simulink model "mracsim"  (R2022a)
settings: Solver=VariableStepAuto  StartTime=0.0  StopTime=100  RelTol=1e-3
undefined symbols (not defined in the file): A, Am, B, Bm, Cm, Dm, Gr, Gx, kr, kx
settings Model: Creator=Joseph  LastModifiedBy=Joseph

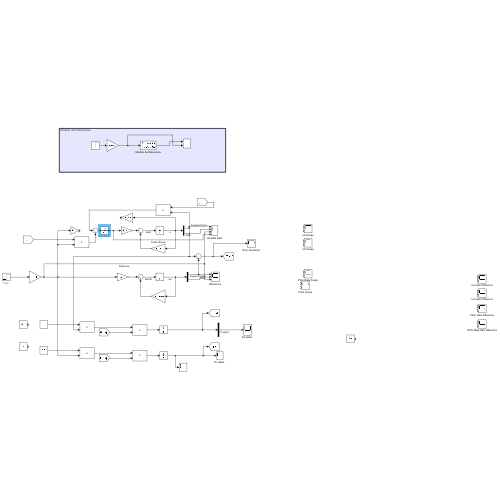
[thumbnail: Simulink's stored preview of the top-level diagram]
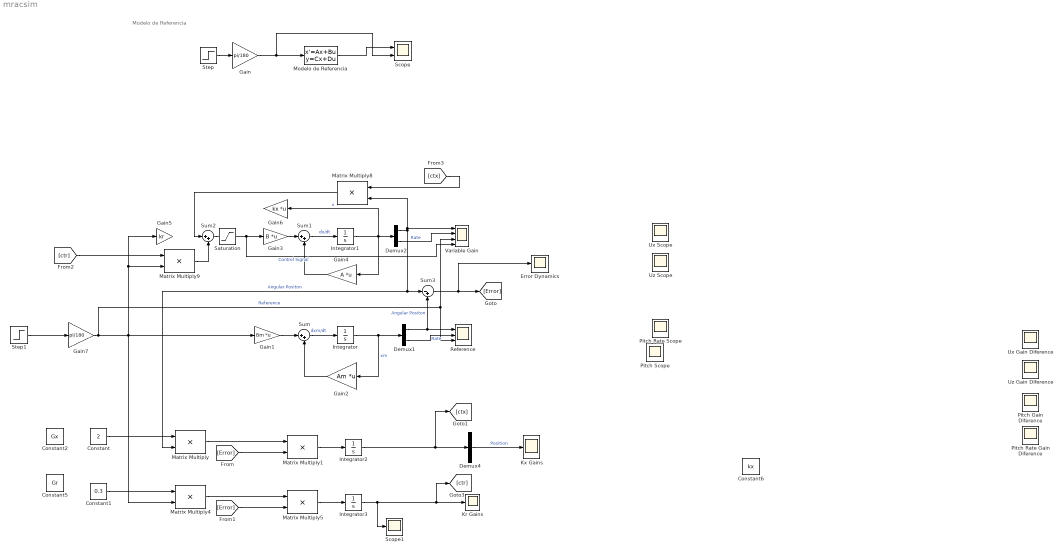
== system mracsim ==
  note: Modelo de Referencia
  Constant : Constant  Value=2
  Constant1 : Constant  Value=0.3
  Constant2 : Constant  Value=Gx
  Constant5 : Constant  Value=Gr
  Constant6 : Constant  Value=kx
  Demux1 : Demux  Outputs=2
  Demux2 : Demux  Outputs=2
  Demux4 : Demux  Outputs=1
  Error Dynamics : Scope
  Gain : Gain  Gain=pi/180
  Gain1 : Gain  Gain=Bm  Multiplication=Matrix(K*u)
  Gain2 : Gain  Gain=Am  Multiplication=Matrix(K*u) (u vector)
  Gain3 : Gain  Gain=B  Multiplication=Matrix(K*u)
  Gain4 : Gain  Gain=A  Multiplication=Matrix(K*u) (u vector)
  Gain5 : Gain  Gain=kr
  Gain6 : Gain  Gain=kx  Multiplication=Matrix(K*u) (u vector)
  Gain7 : Gain  Gain=pi/180
  Integrator{,1..3} (4 alike) : Integrator  ZeroCross=off
  "Kr Gains " : Scope
  "Kx Gains " : Scope
  Matrix Multiply{,1,4..5,8..9} (6 alike) : Product
  Modelo de Referencia : StateSpace  A=Am  B=Bm  C=Cm  D=Dm  InitialCondition=0
  Pitch Gain Diference : Scope  NumInputPorts=2
  Pitch Rate Gain Diference : Scope  NumInputPorts=2
  Pitch Rate Scope : Scope  NumInputPorts=2
  Pitch Scope : Scope  NumInputPorts=2
  Reference : Scope  NumInputPorts=3
  Saturation : Saturate  UpperLimit=9  LowerLimit=0  ZeroCross=off
  Scope : Scope  NumInputPorts=2
  Scope1 : Scope
  Step : Step  Time=0  After=60  SampleTime=0  ZeroCross=off
  Step1 : Step  Time=0  After=60  SampleTime=0  ZeroCross=off
  Sum : Sum  Inputs=|++
  Sum1 : Sum  Inputs=|++
  Sum2 : Sum  Inputs=|++
  Sum3 : Sum  Inputs=|-+
  Ux Gain Diference : Scope  NumInputPorts=2
  Ux Scope : Scope  NumInputPorts=2
  Uz Gain Diference : Scope  NumInputPorts=2
  Uz Scope : Scope  NumInputPorts=2
  Variable Gain : Scope  NumInputPorts=4
  wires:
  Step/1 -> Gain/1
  Gain/1 -> Scope/2, Modelo de Referencia/1
  Modelo de Referencia/1 -> Scope/1
  [ctr] -> Matrix Multiply9/1
  Integrator/1 -> Demux1/1, Gain2/1  "xm"
  [ctx] -> Matrix Multiply8/1
  [Error] -> Matrix Multiply5/2
  Sum2/1 -> Variable Gain/4, Gain3/1  "Control Signal"
  Matrix Multiply4/1 -> Matrix Multiply5/1
  Integrator2/1 -> [ctx], Demux4/1
  Step1/1 -> Gain7/1
  Gain2/1 -> Sum/2
  [Error] -> Matrix Multiply1/2
  Sum/1 -> Integrator/1  "dxm/dt"
  Integrator3/1 -> Scope1/1, [ctr], "Kr Gains "/1
  Integrator1/1 -> Demux2/1, Gain4/1, Gain6/1  "x"
  Gain4/1 -> Sum1/2
  Gain1/1 -> Sum/1
  Matrix Multiply/1 -> Matrix Multiply1/1
  Gain3/1 -> Sum1/1
  Demux4/1 -> "Kx Gains "/1  "Position"
  Sum1/1 -> Integrator1/1  "dx/dt"
  Demux1/2 -> Reference/2  "Rate"
  Demux1/1 -> Sum3/2, Reference/1  "Angular Positon"
  Demux2/1 -> Matrix Multiply8/2, Variable Gain/1, Matrix Multiply/2, Sum3/1  "Angular Positon"
  Sum3/1 -> Error Dynamics/1, [Error]
  Gain7/1 -> Variable Gain/3, Reference/3, Matrix Multiply9/2, Gain5/1, Matrix Multiply4/2, Gain1/1  "Reference"
  Matrix Multiply1/1 -> Integrator2/1
  Matrix Multiply5/1 -> Integrator3/1
  Matrix Multiply8/1 -> Sum2/1
  Matrix Multiply9/1 -> Sum2/2
  Demux2/2 -> Variable Gain/2  "Rate"
  Constant/1 -> Matrix Multiply/1
  Constant1/1 -> Matrix Multiply4/1
